simulink model "controladores_internos_torque_test"  (R2019a)
settings: Solver=VariableStepAuto  StartTime=0.0  StopTime=10.0  RelTol=1e-3
undefined symbols (not defined in the file): sigbuilder_block, T_hm_MAX, T_s2, T_tm_max, tau_hm, tau_tm, w_hm_rated
settings Model: Creator=Facundo  LastModifiedBy=Facundo

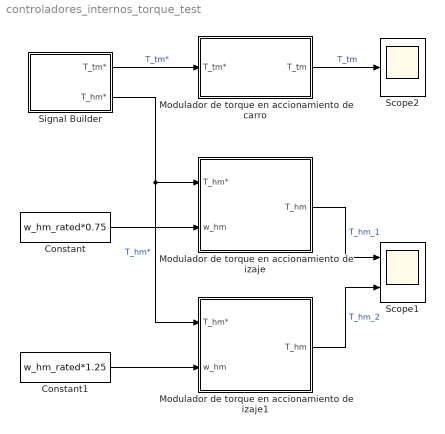
== system controladores_internos_torque_test ==
  Constant : Constant  Value=w_hm_rated*0.75
  Constant1 : Constant  Value=w_hm_rated*1.25
  Modulador de torque en accionamiento de carro : Subsystem
  Modulador de torque en accionamiento de izaje : Subsystem
  Modulador de torque en accionamiento de izaje1 : Subsystem
  Scope1 : Scope  NumInputPorts=2
  Scope2 : Scope
  Signal Builder : Subsystem  Tag=STV Subsys  LoadFcn=sigbuilder_block('load');  StartFcn=sigbuilder_block('start');  StopFcn=sigbuilder_block('stop');  ClipboardFcn=sigbuilder_block('clipboard');  mask(Sigbuilder block){tuvar=[0:10]}
      mask help: Simulink:masks:SigbuilderBlock_MD
      mask init:
      | if ~strcmp(get_param(bdroot(gcbh),'SimulationStatus'),'stopped') tuvar = sigbuilder_block('maskInit'); end
      settings: CopyFcn=sigbuilder_block('copy');  DeleteFcn=sigbuilder_block('delete');  ModelCloseFcn=sigbuilder_block('modelClose');  PreSaveFcn=sigbuilder_block('preSave');  PauseFcn=sigbuilder_block('pause');  ContinueFcn=sigbuilder_block('continue');  NameChangeFcn=sigbuilder_block('namechange');  OpenFcn=sigbuilder_block('open',[-1152 -103.714 1152 564.429 ]);  CloseFcn=sigbuilder_block('close');
      mask Display: plot(0, 0, 100, 100,[2, 2, 32, 32, 2], [68, 8, 8, 68, 68],[32, 2], [38, 38], [32, 19, 2],[53, 60, 44], [32, 17, 17, 2],[16, 16, 31, 31]);txt = getActiveGroup(gcbh);text(2, 100, txt,'verticalAlignment', 'top');
  wires:
  Modulador de torque en accionamiento de carro/1(T_tm) -> Scope2/1  "T_tm"
  Modulador de torque en accionamiento de izaje/1(T_hm) -> Scope1/1  "T_hm_1"
  Signal Builder/2(T_hm*) -> Modulador de torque en accionamiento de izaje1/1(T_hm*), Modulador de torque en accionamiento de izaje/1(T_hm*)  "T_hm*"
  Signal Builder/1(T_tm*) -> Modulador de torque en accionamiento de carro/1(T_tm*)  "T_tm*"
  Constant/1 -> Modulador de torque en accionamiento de izaje/2(w_hm)
  Modulador de torque en accionamiento de izaje1/1(T_hm) -> Scope1/2  "T_hm_2"
  Constant1/1 -> Modulador de torque en accionamiento de izaje1/2(w_hm)

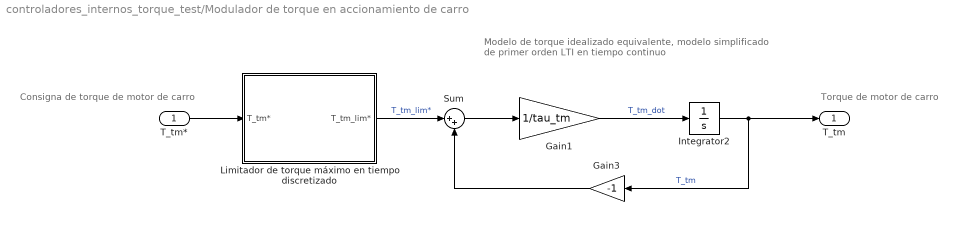
== system controladores_internos_torque_test/Modulador de torque en accionamiento de carro ==
  note: Modelo de torque idealizado equivalente,
      | modelo simplificado de primer orden LTI en tiempo continuo
  note: Consigna de torque de motor de carro
  note: Torque de motor de carro
  T_tm* : Inport
  Gain1 : Gain  Gain=1/tau_tm
  Gain3 : Gain  Gain=-1
  Integrator2 : Integrator
  Limitador de torque máximo en tiempo discretizado : Subsystem
  Sum : Sum  Inputs=|++
  T_tm : Outport
  wires:
  Integrator2/1 -> T_tm/1, Gain3/1  "T_tm"
  Gain3/1 -> Sum/2
  Gain1/1 -> Integrator2/1  "T_tm_dot"
  Sum/1 -> Gain1/1
  Limitador de torque máximo en tiempo discretizado/1(T_tm_lim*) -> Sum/1  "T_tm_lim*"
  T_tm*/1 -> Limitador de torque máximo en tiempo discretizado/1(T_tm*)

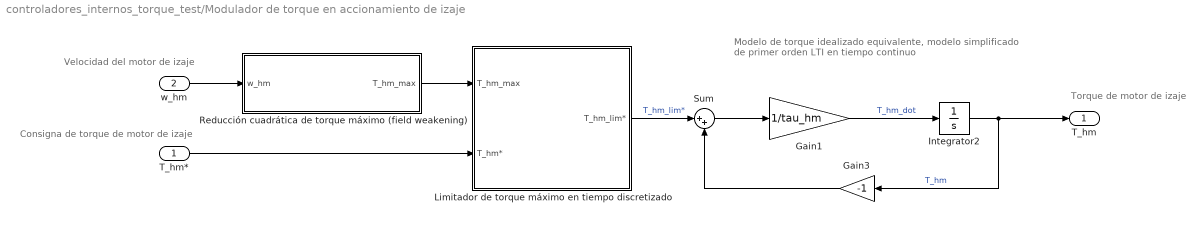
== system controladores_internos_torque_test/Modulador de torque en accionamiento de izaje ==
  note: Modelo de torque idealizado equivalente,
      | modelo simplificado de primer orden LTI en tiempo continuo
  note: Consigna de torque de motor de izaje
  note: Velocidad del motor de izaje
  note: Torque de motor de izaje
  T_hm* : Inport
  w_hm : Inport  Port=2
  Gain1 : Gain  Gain=1/tau_hm
  Gain3 : Gain  Gain=-1
  Integrator2 : Integrator
  Limitador de torque máximo en tiempo discretizado : Subsystem
  Reducción cuadrática de torque máximo (field weakening) : Subsystem
  Sum : Sum  Inputs=|++
  T_hm : Outport
  wires:
  Integrator2/1 -> T_hm/1, Gain3/1  "T_hm"
  Gain3/1 -> Sum/2
  Gain1/1 -> Integrator2/1  "T_hm_dot"
  Sum/1 -> Gain1/1
  Limitador de torque máximo en tiempo discretizado/1(T_hm_lim*) -> Sum/1  "T_hm_lim*"
  Reducción cuadrática de torque máximo (field weakening)/1(T_hm_max) -> Limitador de torque máximo en tiempo discretizado/1(T_hm_max)
  T_hm*/1 -> Limitador de torque máximo en tiempo discretizado/2(T_hm*)
  w_hm/1 -> Reducción cuadrática de torque máximo (field weakening)/1(w_hm)

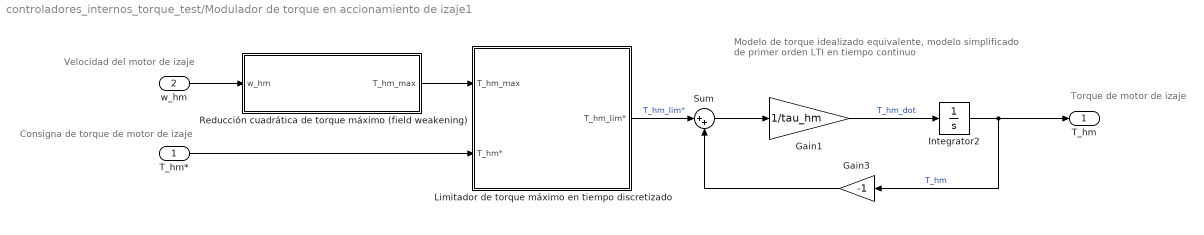
== system controladores_internos_torque_test/Modulador de torque en accionamiento de izaje1 ==
  note: Torque de motor de izaje
  note: Velocidad del motor de izaje
  note: Consigna de torque de motor de izaje
  note: Modelo de torque idealizado equivalente,
      | modelo simplificado de primer orden LTI en tiempo continuo
  T_hm* : Inport
  w_hm : Inport  Port=2
  Gain1 : Gain  Gain=1/tau_hm
  Gain3 : Gain  Gain=-1
  Integrator2 : Integrator
  Limitador de torque máximo en tiempo discretizado : Subsystem
  Reducción cuadrática de torque máximo (field weakening) : Subsystem
  Sum : Sum  Inputs=|++
  T_hm : Outport
  wires:
  w_hm/1 -> Reducción cuadrática de torque máximo (field weakening)/1(w_hm)
  T_hm*/1 -> Limitador de torque máximo en tiempo discretizado/2(T_hm*)
  Reducción cuadrática de torque máximo (field weakening)/1(T_hm_max) -> Limitador de torque máximo en tiempo discretizado/1(T_hm_max)
  Limitador de torque máximo en tiempo discretizado/1(T_hm_lim*) -> Sum/1  "T_hm_lim*"
  Sum/1 -> Gain1/1
  Gain1/1 -> Integrator2/1  "T_hm_dot"
  Gain3/1 -> Sum/2
  Integrator2/1 -> Gain3/1, T_hm/1  "T_hm"

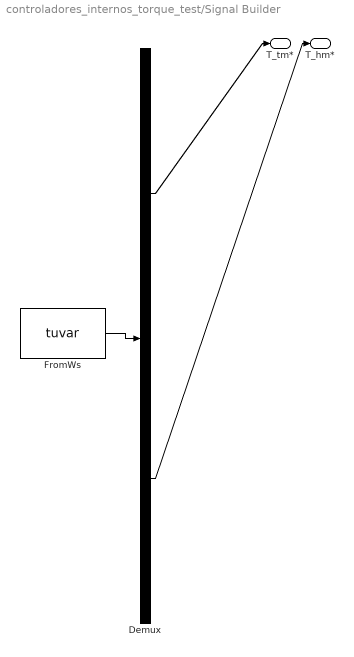
== system controladores_internos_torque_test/Signal Builder ==
  Demux : Demux  Tag=STV Demux  Outputs=2
  FromWs : FromWorkspace  Tag=STV FromWs  VariableName=tuvar  SampleTime=0
      SigBuilderData=|
      | common.afterFinalStr = 'Extrapolate'
      | common.sampleTime = 0
      | dataSet.timeRange = [0 10]
      | dataSet.name = 'Group 1'
      | sbobj.Groups.Name = 'Group 1'
      | sbobj.Groups.Signals(1).Name = 'T_tm*'
      | sbobj.Groups.Signals(1).XData = [0 0.5 10]
      | sbobj.Groups.Signals(1).YData = [0 0 3500]
      | sbobj.Groups.Signals(2).Name = 'T_hm*'
      | sbobj.Groups.Signals(2).XData = [0 0.5 10]
      | sbobj.Groups.Signals(2).YData = [0 0 25000]
  T_tm* : Outport  Tag=STV Outport
  T_hm* : Outport  Tag=STV Outport  Port=2
  wires:
  FromWs/1 -> Demux/1
  Demux/1 -> T_tm*/1
  Demux/2 -> T_hm*/1

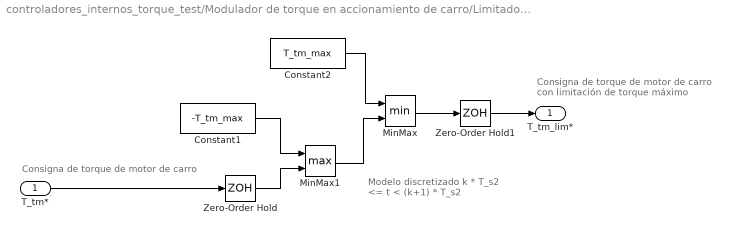
== system controladores_internos_torque_test/Modulador de torque en accionamiento de carro/Limitador de torque máximo en tiempo discretizado ==
  note: Consigna de torque de motor de carro
  note: Consigna de torque de motor de carro
      | con limitación de torque máximo
  note: Modelo discretizado
      | k * T_s2 <= t < (k+1) * T_s2
  T_tm* : Inport
  Constant1 : Constant  Value=-T_tm_max
  Constant2 : Constant  Value=T_tm_max
  MinMax : MinMax  Inputs=2
  MinMax1 : MinMax  Function=max  Inputs=2
  Zero-Order Hold : ZeroOrderHold  SampleTime=T_s2
  Zero-Order Hold1 : ZeroOrderHold  SampleTime=T_s2
  T_tm_lim* : Outport
  wires:
  T_tm*/1 -> Zero-Order Hold/1
  MinMax/1 -> Zero-Order Hold1/1
  Constant1/1 -> MinMax1/1
  MinMax1/1 -> MinMax/2
  Zero-Order Hold/1 -> MinMax1/2
  Zero-Order Hold1/1 -> T_tm_lim*/1
  Constant2/1 -> MinMax/1

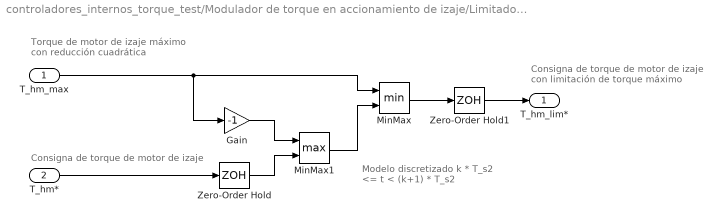
== system controladores_internos_torque_test/Modulador de torque en accionamiento de izaje/Limitador de torque máximo en tiempo discretizado ==
  note: Torque de motor de izaje máximo
      | con reducción cuadrática
  note: Consigna de torque de motor de izaje
  note: Consigna de torque de motor de izaje
      | con limitación de torque máximo
  note: Modelo discretizado
      | k * T_s2 <= t < (k+1) * T_s2
  T_hm_max : Inport
  T_hm* : Inport  Port=2
  Gain : Gain  Gain=-1
  MinMax : MinMax  Inputs=2
  MinMax1 : MinMax  Function=max  Inputs=2
  Zero-Order Hold : ZeroOrderHold  SampleTime=T_s2
  Zero-Order Hold1 : ZeroOrderHold  SampleTime=T_s2
  T_hm_lim* : Outport
  wires:
  T_hm*/1 -> Zero-Order Hold/1
  MinMax/1 -> Zero-Order Hold1/1
  T_hm_max/1 -> MinMax/1, Gain/1
  Gain/1 -> MinMax1/1
  MinMax1/1 -> MinMax/2
  Zero-Order Hold/1 -> MinMax1/2
  Zero-Order Hold1/1 -> T_hm_lim*/1

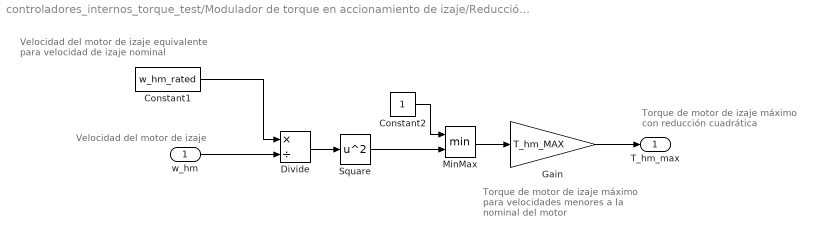
== system controladores_internos_torque_test/Modulador de torque en accionamiento de izaje/Reducción cuadrática de torque máximo (field weakening) ==
  note: Velocidad del motor de izaje
  note: Velocidad del motor de izaje equivalente
      | para velocidad de izaje nominal
  note: Torque de motor de izaje máximo
      | con reducción cuadrática
  note: Torque de motor de izaje
      | máximo para velocidades
      | menores a la nominal del motor
  w_hm : Inport
  Constant1 : Constant  Value=w_hm_rated
  Constant2 : Constant
  Divide : Product  Inputs=*/
  Gain : Gain  Gain=T_hm_MAX
  MinMax : MinMax  Inputs=2
  Square : Math  Operator=square  SaturateOnIntegerOverflow=on
  T_hm_max : Outport
  wires:
  Constant2/1 -> MinMax/1
  MinMax/1 -> Gain/1
  Gain/1 -> T_hm_max/1
  w_hm/1 -> Divide/2
  Constant1/1 -> Divide/1
  Divide/1 -> Square/1
  Square/1 -> MinMax/2

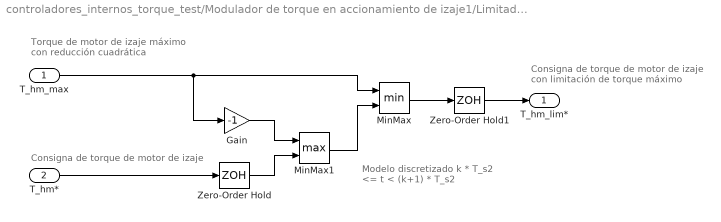
== system controladores_internos_torque_test/Modulador de torque en accionamiento de izaje1/Limitador de torque máximo en tiempo discretizado ==
  note: Modelo discretizado
      | k * T_s2 <= t < (k+1) * T_s2
  note: Consigna de torque de motor de izaje
      | con limitación de torque máximo
  note: Consigna de torque de motor de izaje
  note: Torque de motor de izaje máximo
      | con reducción cuadrática
  T_hm_max : Inport
  T_hm* : Inport  Port=2
  Gain : Gain  Gain=-1
  MinMax : MinMax  Inputs=2
  MinMax1 : MinMax  Function=max  Inputs=2
  Zero-Order Hold : ZeroOrderHold  SampleTime=T_s2
  Zero-Order Hold1 : ZeroOrderHold  SampleTime=T_s2
  T_hm_lim* : Outport
  wires:
  Zero-Order Hold1/1 -> T_hm_lim*/1
  Zero-Order Hold/1 -> MinMax1/2
  MinMax1/1 -> MinMax/2
  Gain/1 -> MinMax1/1
  T_hm_max/1 -> Gain/1, MinMax/1
  MinMax/1 -> Zero-Order Hold1/1
  T_hm*/1 -> Zero-Order Hold/1

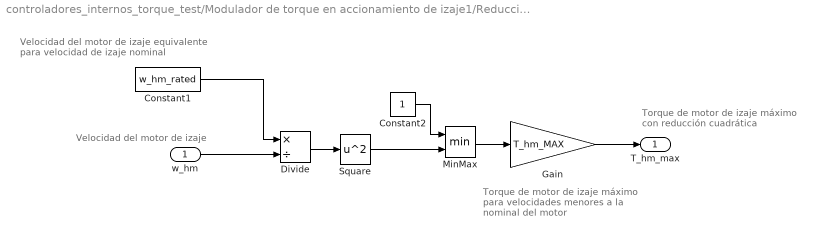
== system controladores_internos_torque_test/Modulador de torque en accionamiento de izaje1/Reducción cuadrática de torque máximo (field weakening) ==
  note: Torque de motor de izaje
      | máximo para velocidades
      | menores a la nominal del motor
  note: Torque de motor de izaje máximo
      | con reducción cuadrática
  note: Velocidad del motor de izaje equivalente
      | para velocidad de izaje nominal
  note: Velocidad del motor de izaje
  w_hm : Inport
  Constant1 : Constant  Value=w_hm_rated
  Constant2 : Constant
  Divide : Product  Inputs=*/
  Gain : Gain  Gain=T_hm_MAX
  MinMax : MinMax  Inputs=2
  Square : Math  Operator=square  SaturateOnIntegerOverflow=on
  T_hm_max : Outport
  wires:
  Square/1 -> MinMax/2
  Divide/1 -> Square/1
  Constant1/1 -> Divide/1
  w_hm/1 -> Divide/2
  Gain/1 -> T_hm_max/1
  MinMax/1 -> Gain/1
  Constant2/1 -> MinMax/1
